simulink model "Hadamard_Ex3"  (R2025a)
settings: Solver=VariableStepAuto  StartTime=0.0  StopTime=10  RelTol=1e-3
undefined symbols (not defined in the file): Correlation_ValidMode, DUT, L, vsva1596, xcvc1702
libraries: aieUtilities x2, aieDSP x1, vmcUtilities x1
settings Model: Creator=sdegala  LastModifiedBy=sdegala
settings ModelReferenceCC: EnableRefExpFcnMdlSchedulingChecks=on
settings RTWCC: GPUComputeCapability=3.5

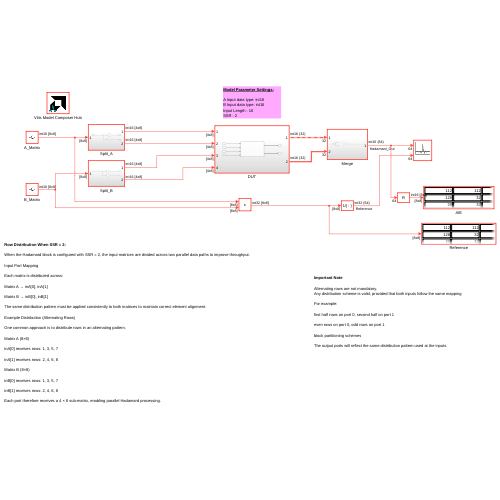
[thumbnail: Simulink's stored preview of the top-level diagram]
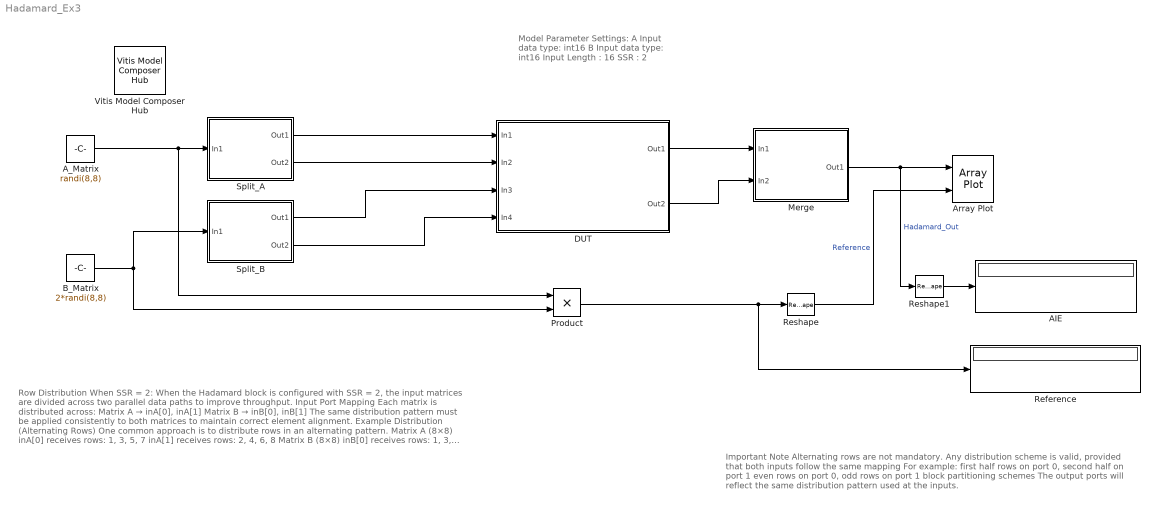
== system Hadamard_Ex3 ==
  note: Important Note
      |
      | Alternating rows are not mandatory.
      | Any distribution scheme is valid, provided that both inputs follow the same mapping
      |
      | For example:
      |
      | first half rows on port 0, second half on port 1
      |
      | even rows on port 0, odd rows on port 1
      |
      | block partitioning schemes
      |
      | The output ports will reflect the same distribution pattern used at the inputs.
  note: Row Distribution When SSR = 2:
      |
      | When the Hadamard block is configured with SSR = 2, the input matrices are divided across two parallel data paths to improve throughput.
      |
      | Input Port Mapping
      |
      | Each matrix is distributed across:
      |
      | Matrix A → inA[0], inA[1]
      |
      | Matrix B → inB[0], inB[1]
      |
      | The same distribution pattern must be applied consistently to both matrices to maintain correct element alignment.
      |
      | Example Distribution (Alternating Rows)
      |
      | One common approach is to distribute rows in an alternating pattern.
      |
      | Matrix A (8×8)
      |
      | inA[0] receives rows: 1, 3, 5, 7
      |
      | inA[1] receives rows: 2, 4, 6, 8
      |
      | Matrix B (8×8)
      |
      | inB[0] receives rows: 1, 3, 5, 7
      |
      | inB[1] receives rows: 2, 4, 6, 8
      |
      | Each port therefore receives a 4 × 8 sub-matrix, enabling parallel Hadamard processing.
  note: Model Parameter Settings:
      |
      | A Input data type: int16
      | B Input data type: int16
      | Input Length : 16
      | SSR : 2
  AIE : Display
  A_Matrix : Constant  Value=randi(8,8)  OutDataTypeStr=int16  SampleTime=1
  Array Plot : ArrayPlot  NumInputPorts=2  WindowPosition=[270.000000,224.000000,800.000000,500.000000,]  Visible=on  ScopeFrameLocation=window  YLimits=[-13.75 143.75]  ShowLegend=on
  B_Matrix : Constant  Value=2*randi(8,8)  OutDataTypeStr=int16  SampleTime=1
  DUT : Subsystem
  Merge : Subsystem
  Product : Product
  Reference : Display
  Reshape : Reshape
  Reshape1 : Reshape  OutputDimensionality=Customize  OutputDimensions=[8,8]
  Split_A : Subsystem
  Split_B : Subsystem
  Vitis Model Composer Hub : vmcUtilities/Vitis Model Composer Hub  Tag=genX  CodeGeneration=off  SubsystemName=DUT  BlockHierPath=Correlation_ValidMode/DUT  SubsystemType=AIENode  StartColumn=1  NumberOfColumns=1  TargetDirectory=./code  exportDesign=off  analyzeDesign=on  validateDesignOnHw=off  ExportType=AI Engines  IpVendor=xilinx.com  IpLibrary=hls  IpVersion=1.0  IpHWLanguage=Verilog  AieCompilerOptions={}  AieSimulatorOptions={}  CreateTestbench=on  TestbenchStackSize=10  RunRtlSim=off  RunCSim=off  RunAieSim=off  AieSimTimeout=50000  RunAieSimProfiling=off  LaunchVitisAnalyzer=off  PlotOutput=off  RunX86Sim=off  X86SimTimeout=10  GenHwImage=off  GenLibadfXo=off  GenHwValidationCode=off  PlatformType=Not Specified  HwSystemType=Baremetal  HwValidationTarget=hw  ProjDevice=xcvc1702-vsva1596-2LP-e-L  ProjDevicePart=xcvc1702-vsva1596-2LP-e-L  AIEType=AIE  SamplePeriod=-1  ClockFrequency=200  DataPathParallelism=1  xilinxfamily=versalaicore  part=xcvc1702  speed=-2LP-e-L  package=vsva1596  directory=./netlist  testbench=off  incr_netlist=off  synthesis_tool=Vivado  clock_wrapper=Clock Enables  dbl_ovrd=According to Block Masks  dcm_input_clock_period=10  sysclk_period=10  simulink_period=1  eval_field=0  IPInfoJsonString="{\"DUTSubsystemName\":\"DUT\",\"AIESubsystem\":{\"SubsystemName\":\"DUT\",\"TargetDirectory\":\"./code\",\"AIEArrayConfig\":\"Use entire AIE array\",\"StartColumn\":\"0\",\"NumberOfColumns\":\"1\"},\"SubsystemTag\":\"AIENode\"}"  LogFileName=/proj/xhdhdstaff5/sdegala/Head1/HEAD/2025_2_work/AIE_BLOCKS_2025_2/code/model_composer.log  NThreads=4  IPConfigFile=/tmp/vmctmp-11198269997411262707/Correlation_ValidMode_ipconfig.json
  wires:
  Product/1 -> Reference/1, Reshape/1
  Reshape/1 -> Array Plot/2  "Reference"
  A_Matrix/1 -> Split_A/1(In1), Product/1
  B_Matrix/1 -> Product/2, Split_B/1(In1)
  Merge/1(Out1) -> Array Plot/1, Reshape1/1  "Hadamard_Out"
  Split_A/1(Out1) -> DUT/1(In1)
  Split_A/2(Out2) -> DUT/2(In2)
  Split_B/1(Out1) -> DUT/3(In3)
  Split_B/2(Out2) -> DUT/4(In4)
  DUT/1(Out1) -> Merge/1(In1)
  DUT/2(Out2) -> Merge/2(In2)
  Reshape1/1 -> AIE/1

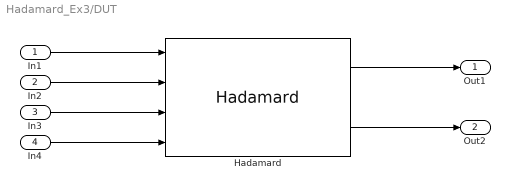
== system Hadamard_Ex3/DUT ==
  In1 : Inport
  In2 : Inport  Port=2
  In3 : Inport  Port=3
  In4 : Inport  Port=4
  Hadamard : aieDSP/Hadamard  AIE_VARIANT=1  TP_API=0  data_type_A=int16  data_type_B=int16  dim_size=64  num_frames=1  shift_output=0  ssr=2  rnd_mode=Floor  sat_mode=None  blockJsonConstraints=[]  blockJsonConstraintsInternal=[]  spec=vmc_hadamard.json  SerializedMaskParamNames=[]  SerializedMaskParamValues=[]  SerializedMaskParamVisibilities=[]  block_type=Hadamard  SerializedMaskParamDataypes=uint|uint|typename|typename|uint|uint|uint|uint|uint|uint  SerializedMaskParamEnumStrArr=0|0|0|0|0|0|0|0|Floor,Ceiling,Round to positive infinity,Round to negative infinity,Round symmetrical to infinity,Round symmetrical to zero,Round convergent to even,Round convergent to odd|None,Saturate,Symmetric  SerializedMaskParamEnumValArr=0|0|0|0|0|0|0|0|0,1,2,3,4,5,6,7|0,1,3  SerializedMaskParamVectorArr=0|0|0|0|0|0|0|0|0|0  SerializedMaskParamKeys=AIE_VARIANT|TP_API|TT_DATA_A|TT_DATA_B|TP_DIM|TP_NUM_FRAMES|TP_SHIFT|TP_SSR|TP_RND|TP_SAT
  Out1 : Outport
  Out2 : Outport  Port=2
  wires:
  In1/1 -> Hadamard/1
  In2/1 -> Hadamard/2
  Hadamard/2 -> Out2/1
  In4/1 -> Hadamard/4
  Hadamard/1 -> Out1/1
  In3/1 -> Hadamard/3

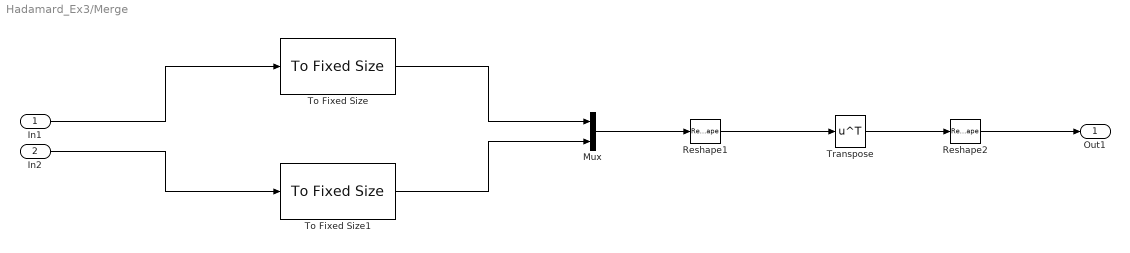
== system Hadamard_Ex3/Merge ==
  In1 : Inport
  In2 : Inport  Port=2
  Mux : Mux  Inputs=2
  Reshape1 : Reshape  OutputDimensionality=Customize  OutputDimensions=[32, 2]
  Reshape2 : Reshape  OutputDimensions=[1, 10]
  To Fixed Size : aieUtilities/To Fixed Size  Mode=Stop simulation when input variable-size signal is not full  OutputSize=Inherit: Same as input  CopyMethod=Buffer samples to form output  HasStatusOutput=on
  To Fixed Size1 : aieUtilities/To Fixed Size  Mode=Stop simulation when input variable-size signal is not full  OutputSize=Inherit: Same as input  CopyMethod=Buffer samples to form output  HasStatusOutput=on
  Transpose : Math  Operator=transpose
  Out1 : Outport
  wires:
  Reshape1/1 -> Transpose/1
  To Fixed Size/1 -> Mux/1
  In1/1 -> To Fixed Size/1
  Mux/1 -> Reshape1/1
  In2/1 -> To Fixed Size1/1
  Transpose/1 -> Reshape2/1
  To Fixed Size1/1 -> Mux/2
  Reshape2/1 -> Out1/1

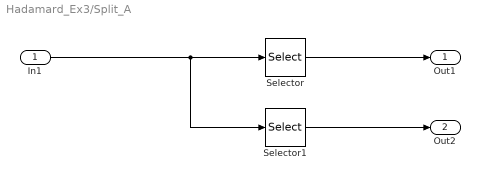
== system Hadamard_Ex3/Split_A ==
  In1 : Inport
  Selector : Selector  NumberOfDimensions=2  InputPortWidth=64  IndexOptions=Index vector (dialog),Index vector (dialog)  Indices=1:2:8,1:8  OutputSizes=1,1
  Selector1 : Selector  NumberOfDimensions=2  InputPortWidth=64  IndexOptions=Index vector (dialog),Index vector (dialog)  Indices=2:2:8,1:8  OutputSizes=1,1
  Out1 : Outport
  Out2 : Outport  Port=2
  wires:
  In1/1 -> Selector/1, Selector1/1
  Selector1/1 -> Out2/1
  Selector/1 -> Out1/1

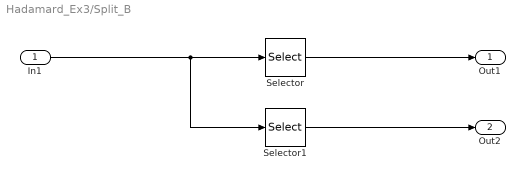
== system Hadamard_Ex3/Split_B ==
  In1 : Inport
  Selector : Selector  NumberOfDimensions=2  InputPortWidth=64  IndexOptions=Index vector (dialog),Index vector (dialog)  Indices=1:2:8,1:8  OutputSizes=1,1
  Selector1 : Selector  NumberOfDimensions=2  InputPortWidth=64  IndexOptions=Index vector (dialog),Index vector (dialog)  Indices=2:2:8,1:8  OutputSizes=1,1
  Out1 : Outport
  Out2 : Outport  Port=2
  wires:
  In1/1 -> Selector/1, Selector1/1
  Selector1/1 -> Out2/1
  Selector/1 -> Out1/1
